simulink model "RemoteCHIL"  (Simulink 8.1)
settings: Solver=ode1  StartTime=0.0  StopTime=inf  FixedStep=Ts  MaxStep=1e-3  RelTol=1e-3
PostLoadFcn:
  | NREL_Mode=3; BANSHEE_init;
InitFcn:
  | NREL_Mode=3; BANSHEE_init;
values from neighbouring files (symbols this model uses):
  F4 = xlsread('F4_relay_nrel.xlsx')    [relay_settings_init.m]
  Ts = 100E-6    (= 0.0001)    [BANSHEE_init.m]    (also in Ghost_init.m)
undefined symbols (not defined in the file or in its folder): Left, Stim, type, V
libraries: simulink x50, relay_modbus_lib x11, simulink_extras x10, rtio_generic_modbus x6, rtlab x5, RMS_lib x4, cables_lib x3, relay_PLL_lib x3, PHIL_lib x2, breaker_lib x2, powerlib_extras x2, relay_ANSI_functions_lib x2
(part 2 of 3)

== system RemoteCHIL/SC_ctrl/TestSeq ==
  TestData : Inport
  Bias : Bias  Bias=[0:-1:-10]*1.1
  Bias1 : Bias  Bias=[0:-1:-2]*1.1
  Bias2 : Bias  Bias=[0:-1:-1]*1.1
  Bias3 : Bias  Bias=[0:-1:-1]*1.1
  Bus Selector : BusSelector  OutputSignals=TestSeq.seq_time,TestSeq.fault,TestSeq.dms,TestSeq.grid,TestSeq.motor,TestSeq.misc
  Bus Selector1 : BusSelector  OutputSignals=loc1,loc2,loc3,loc4,loc5,loc6,gen1,gen2,gen3,pv1,pv2  OutputAsBus=on
  Bus Selector2 : BusSelector  OutputSignals=DisReq,kWEna,PFEna  OutputAsBus=on
  Bus Selector3 : BusSelector  OutputSignals=kWref,PFref
  Bus Selector4 : BusSelector  OutputSignals=Dp,Dq  OutputAsBus=on
  Bus Selector5 : BusSelector  OutputSignals=Hz,Volt  OutputAsBus=on
  Bus Selector6 : BusSelector  OutputSignals=ena1,ena2  OutputAsBus=on
  Bus Selector7 : BusSelector  OutputSignals=cut_grid,mgc_ena  OutputAsBus=on
  Bus Selector8 : BusSelector  OutputSignals=TestSeq.price,TestSeq.pv.insolation1,TestSeq.pv.insolation2  OutputAsBus=on
  Display : Display
  Gain : Gain  Gain=[1/60 1/115000]
  TestSequence : Scope  NumInputPorts=9
      settings: YMin=-5~-5~-5~-5~-5~-5~-5~-5~-5  YMax=5~5~5~5~5~5~5~5~5  Decimation=50
  wires:
  TestData/1 -> Bus Selector8/1, Bus Selector/1
  Bus Selector/1 -> Display/1  "<seq_time>"
  Bus Selector/2 -> Bus Selector1/1  "<fault>"
  Bus Selector1/1 -> Bias/1
  Bias/1 -> TestSequence/1  "flt: loc1-6, gen1-3, ess1-2, pv1-2"
  Bus Selector2/1 -> Bias1/1
  Bias1/1 -> TestSequence/2  "dms: DisReq, kwCmd, PFCmd"
  Bus Selector3/1 -> TestSequence/3  "<kWref>"
  Bus Selector3/2 -> TestSequence/4  "<PFref>"
  Bus Selector4/1 -> TestSequence/5  "Dp, Dq"
  Bus Selector/3 -> Bus Selector3/1, Bus Selector4/1, Bus Selector2/1  "<dms>"
  Bus Selector/4 -> Bus Selector5/1  "<grid>"
  Bus Selector5/1 -> Gain/1
  Gain/1 -> TestSequence/6  "GridPU: Hz/Volt"
  Bus Selector/5 -> Bus Selector6/1  "<motor>"
  Bus Selector6/1 -> Bias2/1
  Bias2/1 -> TestSequence/7  "motor: ena1, ena2"
  Bus Selector/6 -> Bus Selector7/1  "<misc>"
  Bus Selector7/1 -> Bias3/1
  Bias3/1 -> TestSequence/8  "misc: cut_grid, mgc_ena"
  Bus Selector8/1 -> TestSequence/9  "price, pv1, pv2"

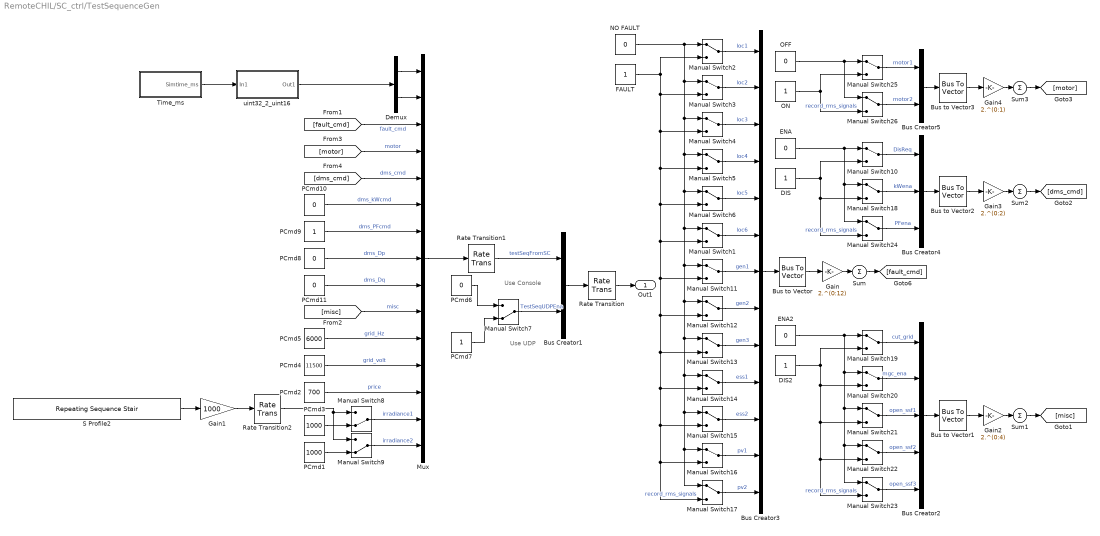
== system RemoteCHIL/SC_ctrl/TestSequenceGen ==
  note: Use Console
  note: Use UDP
  Bus Creator1 : BusCreator  Inputs=2
  Bus Creator2 : BusCreator  Inputs=5
  Bus Creator3 : BusCreator  Inputs=13
  Bus Creator4 : BusCreator  Inputs=3
  Bus Creator5 : BusCreator  Inputs=2
  Bus to Vector{,1..3} (4 alike) : BusToVector
  DIS : Constant
  DIS2 : Constant
  Demux : Demux  Outputs=2
  ENA : Constant  Value=0
  ENA2 : Constant  Value=0
  FAULT : Constant
  Gain : Gain  Gain=2.^(0:12)
  Gain1 : Gain  Gain=1000
  Gain2 : Gain  Gain=2.^(0:4)
  Gain3 : Gain  Gain=2.^(0:2)
  Gain4 : Gain  Gain=2.^(0:1)
  Manual Switch{1..6,10..26} (23 alike) : ManualSwitch
  Manual Switch7 : ManualSwitch  CurrentSetting=0
  Manual Switch8 : ManualSwitch  CurrentSetting=0
  Manual Switch9 : ManualSwitch  CurrentSetting=0
  Mux : Mux  Inputs=15
  NO FAULT : Constant  Value=0
  OFF : Constant  Value=0
  ON : Constant
  PCmd1 : Constant  Value=1000
  PCmd10 : Constant  Value=0
  PCmd11 : Constant  Value=0
  PCmd2 : Constant  Value=700
  PCmd3 : Constant  Value=1000
  PCmd4 : Constant  Value=11500
  PCmd5 : Constant  Value=6000
  PCmd6 : Constant  Value=0  SampleTime=[Stim.Ts Ts]
  PCmd7 : Constant
  PCmd8 : Constant  Value=0
  PCmd9 : Constant
  Rate Transition : RateTransition  Deterministic=off
  Rate Transition1 : RateTransition  Deterministic=off  OutPortSampleTime=1e-2
  Rate Transition2 : RateTransition  Deterministic=off  OutPortSampleTime=1e-2
  S Profile2 : simulink/Sources/Repeating Sequence Stair  OutValues=Stim.PV2.Irradiance  tsamp=[Stim.Ts Ts]  OutMin=[]  OutMax=[]  OutDataTypeStr=Inherit: Inherit via back propagation  OutDataType=fixdt(0,8)  ConRadixGroup=Best Precision: Vector-wise  OutScaling=2^-12
  Sum{,1..3} (4 alike) : Sum  Inputs=+
  Time_ms : Subsystem
  uint32_2_uint16 : Subsystem
      mask Display: disp('uint32_2_uint16');
  Out1 : Outport
  wires:
  Manual Switch4/1 -> Bus Creator3/3  "loc3"
  Manual Switch5/1 -> Bus Creator3/4  "loc4"
  [fault_cmd] -> Mux/3  "fault_cmd"
  Bus Creator3/1 -> Bus to Vector/1
  Manual Switch2/1 -> Bus Creator3/1  "loc1"
  Manual Switch6/1 -> Bus Creator3/5  "loc5"
  Manual Switch3/1 -> Bus Creator3/2  "loc2"
  Manual Switch1/1 -> Bus Creator3/6  "loc6"
  Manual Switch13/1 -> Bus Creator3/9  "gen3"
  Manual Switch14/1 -> Bus Creator3/10  "ess1"
  Manual Switch11/1 -> Bus Creator3/7  "gen1"
  Manual Switch15/1 -> Bus Creator3/11  "ess2"
  Manual Switch12/1 -> Bus Creator3/8  "gen2"
  FAULT/1 -> Manual Switch2/2, Manual Switch1/2, Manual Switch12/2, Manual Switch13/2, Manual Switch14/2, Manual Switch17/2, Manual Switch16/2, Manual Switch15/2, Manual Switch11/2, Manual Switch6/2, Manual Switch5/2, Manual Switch4/2, Manual Switch3/2  "record_rms_signals"
  NO FAULT/1 -> Manual Switch12/1, Manual Switch13/1, Manual Switch14/1, Manual Switch15/1, Manual Switch17/1, Manual Switch16/1, Manual Switch11/1, Manual Switch1/1, Manual Switch6/1, Manual Switch5/1, Manual Switch4/1, Manual Switch3/1, Manual Switch2/1
  Manual Switch16/1 -> Bus Creator3/12  "pv1"
  Manual Switch17/1 -> Bus Creator3/13  "pv2"
  Bus to Vector/1 -> Gain/1
  Gain/1 -> Sum/1
  Sum/1 -> [fault_cmd]
  Mux/1 -> Rate Transition1/1
  Bus Creator1/1 -> Rate Transition/1
  Manual Switch7/1 -> Bus Creator1/2  "TestSeqUDPEna"
  PCmd6/1 -> Manual Switch7/1
  PCmd7/1 -> Manual Switch7/2
  Rate Transition/1 -> Out1/1
  PCmd3/1 -> Manual Switch8/2
  Manual Switch9/1 -> Mux/15  "irradiance2"
  PCmd1/1 -> Manual Switch9/2
  Manual Switch8/1 -> Mux/14  "irradiance1"
  PCmd2/1 -> Mux/13  "price"
  Gain1/1 -> Rate Transition2/1
  Time_ms/1(Simtime_ms) -> uint32_2_uint16/1(In1)
  Demux/1 -> Mux/1
  Demux/2 -> Mux/2
  PCmd4/1 -> Mux/12  "grid_volt"
  PCmd5/1 -> Mux/11  "grid_Hz"
  [misc] -> Mux/10  "misc"
  [motor] -> Mux/4  "motor"
  [dms_cmd] -> Mux/5  "dms_cmd"
  PCmd8/1 -> Mux/8  "dms_Dp"
  PCmd9/1 -> Mux/7  "dms_PFcmd"
  PCmd10/1 -> Mux/6  "dms_kWcmd"
  PCmd11/1 -> Mux/9  "dms_Dq"
  Manual Switch21/1 -> Bus Creator2/3  "open_ssf1"
  Manual Switch22/1 -> Bus Creator2/4  "open_ssf2"
  Bus Creator2/1 -> Bus to Vector1/1
  Manual Switch19/1 -> Bus Creator2/1  "cut_grid"
  Manual Switch23/1 -> Bus Creator2/5  "open_ssf3"
  Manual Switch20/1 -> Bus Creator2/2  "mgc_ena"
  DIS2/1 -> Manual Switch20/2, Manual Switch21/2, Manual Switch22/2, Manual Switch23/2, Manual Switch19/2  "record_rms_signals"
  ENA2/1 -> Manual Switch19/1, Manual Switch20/1, Manual Switch21/1, Manual Switch22/1, Manual Switch23/1
  Bus to Vector1/1 -> Gain2/1
  Gain2/1 -> Sum1/1
  Sum1/1 -> [misc]
  Manual Switch24/1 -> Bus Creator4/3  "PFena"
  Bus Creator4/1 -> Bus to Vector2/1
  Manual Switch10/1 -> Bus Creator4/1  "DisReq"
  Manual Switch18/1 -> Bus Creator4/2  "kWena"
  DIS/1 -> Manual Switch10/2, Manual Switch24/2, Manual Switch18/2  "record_rms_signals"
  ENA/1 -> Manual Switch24/1, Manual Switch18/1, Manual Switch10/1
  Bus to Vector2/1 -> Gain3/1
  Gain3/1 -> Sum2/1
  Sum2/1 -> [dms_cmd]
  Bus Creator5/1 -> Bus to Vector3/1
  Manual Switch25/1 -> Bus Creator5/1  "motor1"
  Manual Switch26/1 -> Bus Creator5/2  "motor2"
  ON/1 -> Manual Switch26/2, Manual Switch25/2  "record_rms_signals"
  OFF/1 -> Manual Switch25/1, Manual Switch26/1
  Bus to Vector3/1 -> Gain4/1
  Gain4/1 -> Sum3/1
  Sum3/1 -> [motor]
  S Profile2/1 -> Gain1/1
  uint32_2_uint16/1(Out1) -> Demux/1
  Rate Transition1/1 -> Bus Creator1/1  "testSeqFromSC"
  Rate Transition2/1 -> Manual Switch9/1, Manual Switch8/1

== system RemoteCHIL/SS_F4_RELAY_HOUSING/BESS_data ==
  note: 0 .... 10000
      | 0 ... 100%
  Bus Selector1 : BusSelector  OutputSignals=Battery.SoC
  Bus Selector9 : BusSelector  OutputSignals=ESS_DATA
  Constant2 : Constant  Value=0
  Mux : Mux  Inputs=2
  Scale_SoC : Gain  Gain=100
  Out1 : Outport
  wires:
  Scale_SoC/1 -> Out1/1
  [F4_MS_IN] -> Bus Selector9/1
  Bus Selector9/1 -> Bus Selector1/1  "<ESS_DATA>"
  Bus Selector1/1 -> Mux/2  "<SoC>"
  Constant2/1 -> Mux/1
  Mux/1 -> Scale_SoC/1

== system RemoteCHIL/SS_F4_RELAY_HOUSING/DieselData ==
  Bus Selector : BusSelector  OutputSignals=GEN3_DATA.gen.gal_per_hr,GEN3_DATA.cb.relay_out.m.Vpu
  Constant1 : Constant  Value=0
  Constant4 : Constant  Value=0
  Mux : Mux
  scale_diesel1 : Gain  Gain=100
  scale_diesel2 : Gain  Gain=100
  Out2 : Outport
  wires:
  [F4_MS_IN] -> Bus Selector/1
  Bus Selector/1 -> scale_diesel1/1  "<gal_per_hr>"
  scale_diesel1/1 -> Mux/2
  Constant4/1 -> Mux/1
  Mux/1 -> Out2/1
  scale_diesel2/1 -> Mux/4
  Bus Selector/2 -> scale_diesel2/1  "<Vpu>"
  Constant1/1 -> Mux/3

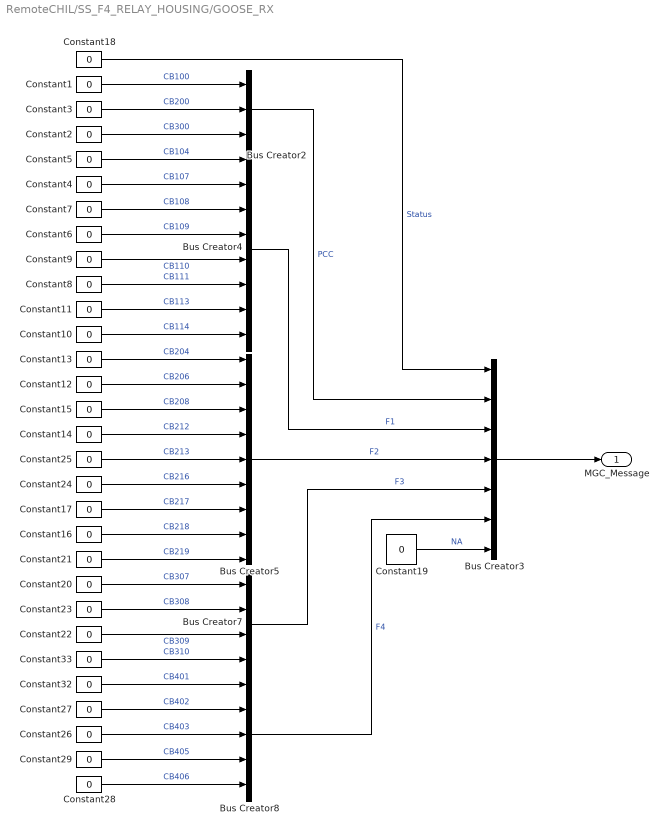
== system RemoteCHIL/SS_F4_RELAY_HOUSING/GOOSE_RX  ==
  Bus Creator2 : BusCreator  Inputs=3
  Bus Creator3 : BusCreator  Inputs=7
  Bus Creator4 : BusCreator  Inputs=8
  Bus Creator5 : BusCreator  Inputs=9
  Bus Creator7 : BusCreator
  Bus Creator8 : BusCreator  Inputs=5
  Constant{1..29,32..33} (31 alike) : Constant  Value=0
  MGC_Message : Outport
  wires:
  Constant18/1 -> Bus Creator3/1  "Status"
  Bus Creator3/1 -> MGC_Message/1
  Constant1/1 -> Bus Creator2/1  "CB100"
  Constant3/1 -> Bus Creator2/2  "CB200"
  Constant2/1 -> Bus Creator2/3  "CB300"
  Bus Creator2/1 -> Bus Creator3/2  "PCC"
  Constant7/1 -> Bus Creator4/3  "CB108"
  Constant6/1 -> Bus Creator4/4  "CB109"
  Constant4/1 -> Bus Creator4/2  "CB107"
  Constant9/1 -> Bus Creator4/5  "CB110"
  Constant5/1 -> Bus Creator4/1  "CB104"
  Constant8/1 -> Bus Creator4/6  "CB111"
  Constant11/1 -> Bus Creator4/7  "CB113"
  Constant10/1 -> Bus Creator4/8  "CB114"
  Bus Creator4/1 -> Bus Creator3/3  "F1"
  Constant21/1 -> Bus Creator5/9  "CB219"
  Constant24/1 -> Bus Creator5/6  "CB216"
  Constant17/1 -> Bus Creator5/7  "CB217"
  Constant25/1 -> Bus Creator5/5  "CB213"
  Constant16/1 -> Bus Creator5/8  "CB218"
  Constant15/1 -> Bus Creator5/3  "CB208"
  Constant13/1 -> Bus Creator5/1  "CB204"
  Constant14/1 -> Bus Creator5/4  "CB212"
  Constant12/1 -> Bus Creator5/2  "CB206"
  Bus Creator5/1 -> Bus Creator3/4  "F2"
  Bus Creator8/1 -> Bus Creator3/6  "F4"
  Constant28/1 -> Bus Creator8/5  "CB406"
  Constant26/1 -> Bus Creator8/3  "CB403"
  Bus Creator7/1 -> Bus Creator3/5  "F3"
  Constant33/1 -> Bus Creator7/4  "CB310"
  Constant22/1 -> Bus Creator7/3  "CB309"
  Constant23/1 -> Bus Creator7/2  "CB308"
  Constant20/1 -> Bus Creator7/1  "CB307"
  Constant19/1 -> Bus Creator3/7  "NA"
  Constant29/1 -> Bus Creator8/4  "CB405"
  Constant27/1 -> Bus Creator8/2  "CB402"
  Constant32/1 -> Bus Creator8/1  "CB401"

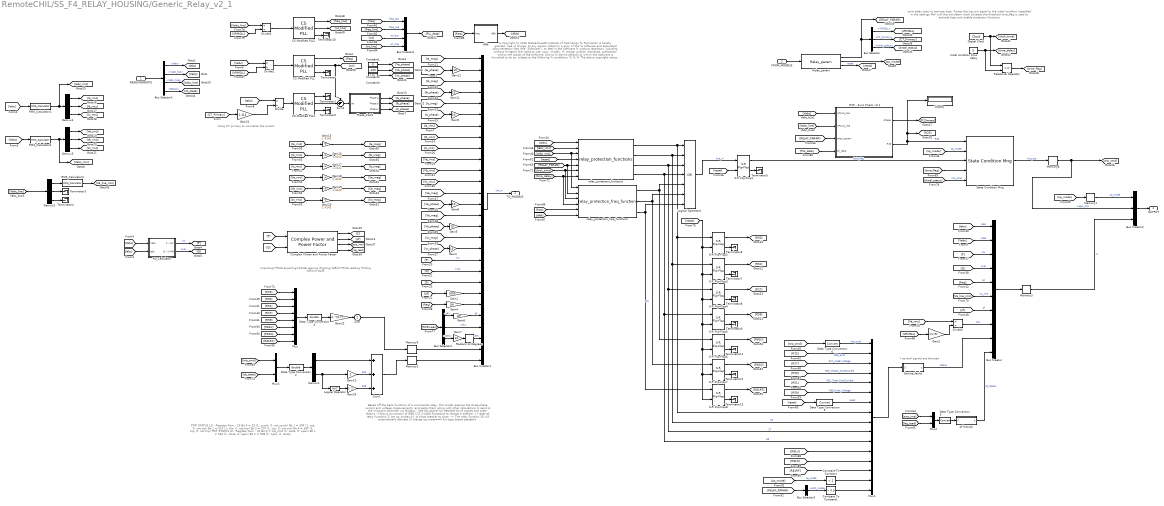
== system RemoteCHIL/SS_F4_RELAY_HOUSING/Generic_Relay_v2_1 ==
  note: time delay [sec] to activate logic. Forces the trip_out signal to the initial condition
      | (specified in the settings file) until the simulation clock exceeds the threshold
      |
      | time_flag is used to activate logic and enable protection functions
  note: Based off the basic functions of a commercial relay, this model receives
      | the three-phase current and voltage measurements, and packs
      | them along with other calculations to send to the microgrid
      | controller via Modbus
      |
      | - See HIL packet for detailed list of signals and scale factors
      | - Follows convention of IEEE C37.2-2008
      |
      | Procedure to reclose a breaker:
      | 1) reset all relay functions
      | 2) set op_mode==1 to force breaker to close
      |    --> The relay function 25 will automatically activate
      | 3) change op_mode==0 for logic based operation
  note: TRIP STATUS LO - Register Num.: 23
      | Bit 0 = 25  (1: synch, 0: not synch)
      | Bit 1 = 50P (1: trip, 0: not trip)
      | Bit 2 = 51P (1: trip, 0: not trip)
      | Bit 3 = 27P (1: trip, 0: not trip)
      | Bit 4 = 59P (1: trip, 0: not trip)
      |
      | TRIP STATUS HI - Register Num.: 24
      | Bit 0 = trip_cmd  (1: close, 0: open)
      | Bit 1 = 52A (1: close, 0: open)
      | Bit 2 = 52B (1: open, 0: close)
  note: Using CT primary to normalize the current.
  note: * several signals are bitwised
  note: Importing=TRUE
      | Exporting=FALSE
      |
      | Lagging (Pushing VARs)=TRUE
      | Leading (Pulling VARs)=FALSE
  note: % Copyright (c) 2016 Massachusetts Institute of Technology
      | % Permission is hereby granted, free of charge, to any person obtaining a copy of this
      | % software and associated documentation files (the "Software"), to deal in the Software
      | % without restriction, including without limitation the rights to use, copy, modify,
      | % merge, publish, distribute, sublicense, and/or sell copies of the Software, and to
      | % permit persons to whom the Software is furnished to do so, subject to the following
      | % conditions:
      | %
      | %
      | % The above copyright notice and this permission notice shall be included in
      | % all copies or substantial portions of the Software.
      | %
      | % THE SOFTWARE IS PROVIDED "AS IS", WITHOUT WARRANTY OF ANY KIND, EXPRESS OR IMPLIED,
      | % INCLUDING BUT NOT LIMITED TO THE WARRANTIES OF MERCHANTABILITY, FITNESS FOR A
      | % PARTICULAR PURPOSE AND NONINFRINGEMENT. IN NO EVENT SHALL THE AUTHORS OR COPYRIGHT
      | % HOLDERS BE LIABLE FOR ANY CLAIM, DAMAGES OR OTHER LIABILITY, WHETHER IN AN ACTION
      | % OF CONTRACT, TORT OR OTHERWISE, ARISING FROM, OUT OF OR IN CONNECTION WITH THE
      | % SOFTWARE OR THE USE OR OTHER DEALINGS IN THE SOFTWARE.
      | %
      | %
      | %%
  MEASUREMENTS : Inport
  FROM_MODBUS : Inport  Port=2
  Bus Creator : BusCreator  Inputs=10
  Bus Creator1 : BusCreator  Inputs=28
  Bus Creator2 : BusCreator  Inputs=3
  Bus Creator3 : BusCreator
  Bus Selector : BusSelector  OutputSignals=VRMSLL,CT_primary,Initial_status
  Bus Selector1 : BusSelector  OutputSignals=Iabc,Vabc_bus,Vabc_line,Status
  Bus Selector2 : BusSelector  OutputSignals=dF,dV,dWt
  Bus Selector3 : BusSelector  OutputSignals=prot_mode
  CS Modified PLL : relay_PLL_lib/CS Modified PLL  Flim=[55 66]  Par_Init=[0 60]  ParK=[ 180 3200 1 ]  Ts=Ts  AGC=off
  CS Modified PLL1 : relay_PLL_lib/CS Modified PLL  Flim=[55 66]  Par_Init=[0 60]  ParK=[ 180 3200 1 ]  Ts=Ts  AGC=off
  CS Modified PLL2 : relay_PLL_lib/CS Modified PLL  Flim=[55 66]  Par_Init=[0 60]  ParK=[ 180 3200 1 ]  Ts=Ts  AGC=off
  Compare To Constant : simulink/Logic and Bit Operations/Compare To Constant  relop=<  const=2  OutDataTypeStr=boolean
  Compare To Constant1 : simulink/Logic and Bit Operations/Compare To Constant  relop=>  const=0.5  OutDataTypeStr=boolean
  Complex Power and Power Factor : relay_PQSPF_lib/Complex Power and Power Factor
  Constant1 : Constant  Value=0
  Constant2 : Constant  Value=-120
  Constant3 : Constant  Value=120
  Data Type Conversion2 : DataTypeConversion  OutDataTypeStr=double
  Data Type Conversion3 : DataTypeConversion
  Data Type Conversion4 : DataTypeConversion  OutDataTypeStr=double
  Data Type Conversion5 : DataTypeConversion
  Data Type Conversion6 : DataTypeConversion
  Demux1 : Demux  Outputs=2
  Demux3 : Demux  Outputs=3
  Demux4 : Demux  Outputs=3
  Demux5 : Demux  Outputs=3
  Digital Clock : DigitalClock  SampleTime=Ts
  Display : Display
  Divide{,1..3} (4 alike) : Product  Inputs=*/
  Gain1 : Gain  Gain=1000
  Gain{3,5,7..9,11..12} (7 alike) : Gain  Gain=10
  Gain13 : Gain  Gain=2
  Gain{15..20} (6 alike) : Gain  Gain=1.4142
  Gain2 : Gain  Gain=1/1.732
  Gain21 : Gain  Gain=1.414
  Gain23 : Gain  Gain=2.^[0:7]
  Gain24 : Gain  Gain=2^2
  Gain4 : Gain  Gain=100
  Gain6 : Gain  Gain=100
  Logical Operator : Logic  Operator=NOT  AllPortsSameDT=off  OutDataTypeStr=boolean
  Logical Operator4 : Logic  Operator=OR  Inputs=7  AllPortsSameDT=off  OutDataTypeStr=boolean
  Memory{1..3,8..9} (5 alike) : Memory
  Mux : Mux  Inputs=8
  Mux1 : Mux  Inputs=16
  Mux2 : Mux  Inputs=2
  Mux3 : Mux  Inputs=2
  PQ_Calculator : Subsystem
  Phase_Calc1 : Subsystem
  R25 - Sync Check v0.1 : Subsystem  AncestorBlock=relay_ANSI_F25_lib/R25 - Sync Check v0.1  mask(Relay synch check){Ts=Ts}
      mask prompts: Ts "Sampling Time [Sec]"
      mask help:
      | This block checks if the the specified conditions for breaker reclosing
      | are met at both terminals of the circuit breaker. This synch check is
      | intended for use in bus-ties, and service lines.
      |
      | The input bus with the relay parameters should be ordered as follows:
      | 1) VRMSLL
      | 2) IOC
      | 3) TOC
      | 4) dV_threshold
      | 5) angle_threshold
      | 6) dF_threshold
  RMS_Calculator1 : RMS_lib/RMS_Calculator  Ts=Ts
  RMS_Calculator2 : RMS_lib/RMS_Calculator  Ts=Ts
  RMS_Calculator3 : RMS_lib/RMS_Calculator  Ts=Ts
  Radians to Degrees : simulink_extras/Transformations/Radians to Degrees
  Relational Operator : RelationalOperator  OutDataTypeStr=boolean
  Relay_param : relay_mgc_cmd_lib/Relay_param  relay_settings=relay_settings
  S-R Flip-Flop{1..8} (8 alike) : simulink_extras/Flip Flops/S-R Flip-Flop  initial_condition=0
  State Condition Mng : relay_tripOutMng_lib/State Condition Mng
  Sum : Sum  Inputs=+
  Sum1 : Sum  Inputs=+++
  Sum2 : Sum  Inputs=-+|
  Terminator{,1..13} (14 alike) : Terminator
  bitwise_faults : Subsystem
  dfdt : Subsystem
  initial condition time delay : Constant  Value=5
  pf bitwise : Subsystem
  relay_protection_freq_functions : relay_ANSI_functions_lib/relay_protection_freq_functions  Ts=Ts
  relay_protection_functions : relay_ANSI_functions_lib/relay_protection_functions  Ts=Ts
  OUTPUT : Outport
  TO_MODBUS : Outport  Port=2
  wires:
  Logical Operator4/1 -> S-R Flip-Flop1/1  "trip_in"
  [reset] -> S-R Flip-Flop1/2
  S-R Flip-Flop1/2 -> Terminator5/1
  Demux1/2 -> Gain13/1, Logical Operator/1
  Gain24/1 -> Sum1/3  "52B"
  [cb_state] -> Mux3/2
  [trip_cmd] -> Mux3/1
  Data Type Conversion2/1 -> Demux1/1
  Demux1/1 -> Sum1/1
  Gain13/1 -> Sum1/2  "52A"
  Mux3/1 -> Data Type Conversion2/1
  [R59] -> Mux/5
  [R27] -> Mux/4
  [R51] -> Mux/3
  [R50] -> Mux/2
  [R25] -> Mux/1
  Bus Selector1/4 -> [cb_state]  "<Status>"
  State Condition Mng/1 -> Memory8/1  "trip_out"
  Demux5/3 -> [Vc_rms]
  Demux5/2 -> [Vb_rms]
  Demux5/1 -> [Va_rms]
  Demux4/1 -> [Ia_rms]
  Demux4/2 -> [Ib_rms]
  Demux4/3 -> [Ic_rms]
  RMS_Calculator2/1 -> [Vabc_rms], Demux5/1
  RMS_Calculator1/1 -> [Iabc_rms], Demux4/1
  [Vabc] -> RMS_Calculator2/1
  [Iabc] -> RMS_Calculator1/1
  PQ_Calculator/2(Q - kVAR) -> [Q]  "kvar"
  PQ_Calculator/1(P - kW) -> [P]  "kw"
  [Iabc] -> PQ_Calculator/2(Iabc)
  [Vabc] -> PQ_Calculator/1(Vabc)
  [Iabc] -> Bus Creator/1  "Iabc"
  [Vabc] -> Bus Creator/2  "Vabc"
  FROM_MODBUS/1 -> Relay_param/1
  Bus Creator1/1 -> TO_MODBUS/1  "sm_in"
  [freq] -> Gain4/1
  [pf] -> Gain1/1
  [P] -> Bus Creator/3  "kw"
  [Q] -> Bus Creator/4  "kvar"
  Constant1/1 -> [Va_phase]
  Constant2/1 -> [Vb_phase]
  Constant3/1 -> [Vc_phase]
  [Iabc] -> Divide/1
  Phase_Calc1/1(Phase a) -> [Ia_phase]
  Phase_Calc1/2(Phase b) -> [Ib_phase]
  Phase_Calc1/3(Phase c) -> [Ic_phase]
  Divide/1 -> CS Modified PLL1/1
  [CT_Primary] -> Gain21/1
  [Vc_phase] -> Gain3/1
  [Vb_phase] -> Gain5/1
  [Va_phase] -> Gain8/1
  [Ic_phase] -> Gain9/1
  [Ib_phase] -> Gain11/1
  [Ia_phase] -> Gain12/1
  Sum1/1 -> Memory2/1
  Sum/1 -> Memory9/1
  relay_protection_functions/2 -> Mux1/9, S-R Flip-Flop3/1, Logical Operator4/2  "51"
  Mux/1 -> Data Type Conversion4/1
  Data Type Conversion4/1 -> Gain23/1
  Memory9/1 -> Bus Creator1/27
  Memory2/1 -> Bus Creator1/28
  [op_mode] -> Memory1/1
  Memory8/1 -> [trip_cmd], Bus Creator2/2  "Logic_trip"
  R25 - Sync Check v0.1/2(R25) -> Display/1, [R25], State Condition Mng/1  "R25"
  [op_mode] -> State Condition Mng/2  "op_mode"
  S-R Flip-Flop1/1 -> State Condition Mng/3  "fault_flag"
  CS Modified PLL1/2 -> Sum2/2
  CS Modified PLL/1 -> [freq]
  CS Modified PLL/2 -> [wt], Sum2/1
  CS Modified PLL1/1 -> Terminator1/1
  CS Modified PLL1/3 -> Terminator2/1
  CS Modified PLL/3 -> Terminator/1
  [freq] -> Bus Creator/5  "Hz"
  [Va_line_rms] -> Bus Creator/6  "Va_rms"
  [pf] -> Bus Creator/7  "pf"
  [Ia_mag] -> Bus Creator1/1
  Gain12/1 -> Bus Creator1/2
  [Ib_mag] -> Bus Creator1/3
  Gain11/1 -> Bus Creator1/4
  [Ic_mag] -> Bus Creator1/5
  Gain9/1 -> Bus Creator1/6
  [Ia_rms] -> Bus Creator1/7
  [Ib_rms] -> Bus Creator1/8
  [Ic_rms] -> Bus Creator1/9
  [Va_rms] -> Bus Creator1/10
  [Vb_rms] -> Bus Creator1/11
  [Vc_rms] -> Bus Creator1/12
  [Va_mag] -> Bus Creator1/13
  Gain8/1 -> Bus Creator1/14
  [Vb_mag] -> Bus Creator1/15
  Gain5/1 -> Bus Creator1/16
  [Vc_mag] -> Bus Creator1/17
  Gain3/1 -> Bus Creator1/18
  Gain1/1 -> Bus Creator1/22
  Gain4/1 -> Bus Creator1/23
  [Vabc] -> R25 - Sync Check v0.1/1(VPKLN_bus)
  [Ia_rms] -> Gain15/1
  [Ib_rms] -> Gain16/1
  [Ic_rms] -> Gain17/1
  [Va_rms] -> Gain18/1
  [Vb_rms] -> Gain19/1
  [Vc_rms] -> Gain20/1
  Gain20/1 -> [Vc_mag]
  Gain19/1 -> [Vb_mag]
  Gain18/1 -> [Va_mag]
  Gain17/1 -> [Ic_mag]
  Gain16/1 -> [Ib_mag]
  Gain15/1 -> [Ia_mag]
  Divide2/1 -> Bus Creator/8  "Vpu"
  relay_protection_functions/3 -> Mux1/10, S-R Flip-Flop4/1, Logical Operator4/3  "27"
  relay_protection_functions/4 -> Mux1/11, S-R Flip-Flop5/1, Logical Operator4/4  "59"
  Mux1/1 -> bitwise_faults/1(S)
  bitwise_faults/1(s) -> Bus Creator/9  "status"
  [reset] -> Data Type Conversion5/1
  [trip_cmd] -> Data Type Conversion6/1
  [R25] -> Mux1/2  "R25_Sync"
  [R27] -> Mux1/3  "R27_Under Voltage"
  [R50] -> Mux1/4  "R50_Instant_OverCurrent"
  [R51] -> Mux1/5  "R51_Time_OverCurrent"
  [R59] -> Mux1/6  "R59_Over_Voltage"
  Data Type Conversion5/1 -> Mux1/7  "reset"
  Data Type Conversion6/1 -> Mux1/1  "trip_cmd"
  [Vabc_line] -> R25 - Sync Check v0.1/2(VPKLN_line)
  Bus Selector1/1 -> [Iabc]  "<Iabc>"
  Bus Selector1/2 -> [Vabc]  "<Vabc_bus>"
  Bus Selector1/3 -> [Vabc_line]  "<Vabc_line>"
  MEASUREMENTS/1 -> Bus Selector1/1
  Bus Creator/1 -> Memory3/1
  Memory1/1 -> Bus Creator2/1  "op_mode"
  Bus Creator2/1 -> OUTPUT/1
  [P] -> Complex Power and Power Factor/1
  [Q] -> Complex Power and Power Factor/2
  Complex Power and Power Factor/1 -> [S]
  Complex Power and Power Factor/2 -> [pf]
  Complex Power and Power Factor/3 -> [exp_imp]
  Complex Power and Power Factor/4 -> [lag_lead]
  Mux2/1 -> Data Type Conversion3/1
  pf bitwise/1(s) -> Bus Creator/10  "pf_states"
  [exp_imp] -> Mux2/1
  [lag_lead] -> Mux2/2
  Memory3/1 -> Bus Creator2/3  "m"
  Data Type Conversion3/1 -> pf bitwise/1(S)
  Bus Selector/2 -> [CT_Primary]  "<CT_primary>"
  Relay_param/1 -> [RELAY_PARAM], Bus Selector/1
  [reset] -> relay_protection_functions/4
  [Iabc_rms] -> relay_protection_functions/2
  [Vabc_rms] -> relay_protection_functions/3, relay_protection_freq_functions/1
  [Iabc] -> relay_protection_functions/1
  [RELAY_PARAM] -> relay_protection_functions/5, relay_protection_freq_functions/2
  [RELAY_PARAM] -> R25 - Sync Check v0.1/3(relay_param)
  Bus Selector/1 -> [VRMSLL]  "<VRMSLL>"
  [Vabc] -> Divide1/1
  Divide1/1 -> CS Modified PLL/1
  [VRMSLL] -> Divide1/2
  [VRMSLL] -> Gain2/1
  [Va_rms] -> Divide2/1
  Relay_param/2 -> [op_mode]
  Gain21/1 -> Divide/2
  Digital Clock/1 -> Relational Operator/1, [clock_time]
  [time_flag] -> State Condition Mng/4
  initial condition time delay/1 -> Relational Operator/2, [time_delay]
  Relay_param/3 -> [reset]  "reset"
  [clock_time] -> relay_protection_functions/6, relay_protection_freq_functions/3
  [time_delay] -> relay_protection_functions/7, relay_protection_freq_functions/4
  Bus Selector/3 -> [Initial_status]  "<Initial_status>"
  [Initial_status] -> State Condition Mng/5  "init_cond"
  Logical Operator/1 -> Gain24/1
  Gain2/1 -> Divide2/2
  Demux3/1 -> RMS_Calculator3/1
  Demux3/2 -> Terminator3/1
  Demux3/3 -> Terminator4/1
  Relational Operator/1 -> [time_flag]
  [Vabc_line] -> Demux3/1
  RMS_Calculator3/1 -> [Va_line_rms]
  S-R Flip-Flop2/2 -> Terminator6/1
  S-R Flip-Flop3/2 -> Terminator7/1
  S-R Flip-Flop4/2 -> Terminator8/1
  S-R Flip-Flop5/2 -> Terminator9/1
  S-R Flip-Flop5/1 -> [R59]
  S-R Flip-Flop4/1 -> [R27]
  S-R Flip-Flop3/1 -> [R51]
  S-R Flip-Flop2/1 -> [R50]
  Sum2/1 -> Phase_Calc1/1(wt)
  [P] -> Bus Creator1/19  "kw"
  [Q] -> Bus Creator1/20  "kvar"
  [S] -> Bus Creator1/21
  relay_protection_functions/1 -> Mux1/8, S-R Flip-Flop2/1, Logical Operator4/1
  R25 - Sync Check v0.1/1(dMeas) -> [R25meas]
  [R25meas] -> Bus Selector2/1
  Bus Selector2/2 -> Bus Creator1/25  "<dV>"
  Bus Selector2/1 -> Gain6/1  "<dF>"
  Bus Selector2/3 -> Gain7/1  "<dWt>"
  Gain6/1 -> Bus Creator1/24  "dF"
  Gain7/1 -> Radians to Degrees/1
  Radians to Degrees/1 -> Bus Creator1/26  "dWt"
  [Vabc_line] -> Divide3/1
  [VRMSLL] -> Divide3/2
  Divide3/1 -> CS Modified PLL2/1
  CS Modified PLL2/1 -> [freq_line]
  CS Modified PLL2/2 -> [wt_line]
  CS Modified PLL2/3 -> Terminator10/1
  [PLL_data] -> R25 - Sync Check v0.1/4(pll_data)
  Bus Creator3/1 -> [PLL_data]
  [freq] -> Bus Creator3/1  "freq_bus"
  [freq_line] -> Bus Creator3/2  "freq_line"
  [wt] -> Bus Creator3/3  "wt_bus"
  [wt_line] -> Bus Creator3/4  "wt_line"
  [freq] -> dfdt/1(freq)
  dfdt/1(dfdt) -> [dfdt]
  [freq] -> relay_protection_freq_functions/5
  [dfdt] -> relay_protection_freq_functions/6
  relay_protection_freq_functions/3 -> S-R Flip-Flop8/1, Logical Operator4/7  "51"
  [reset] -> S-R Flip-Flop8/2, S-R Flip-Flop7/2, S-R Flip-Flop6/2, S-R Flip-Flop5/2, S-R Flip-Flop4/2, S-R Flip-Flop3/2, S-R Flip-Flop2/2
  S-R Flip-Flop6/2 -> Terminator11/1
  S-R Flip-Flop7/2 -> Terminator12/1
  S-R Flip-Flop8/2 -> Terminator13/1
  S-R Flip-Flop8/1 -> [R81RF]
  S-R Flip-Flop7/1 -> [R81O]
  S-R Flip-Flop6/1 -> [R81U]
  relay_protection_freq_functions/1 -> S-R Flip-Flop6/1, Logical Operator4/5
  relay_protection_freq_functions/2 -> Logical Operator4/6, S-R Flip-Flop7/1
  [R81U] -> Mux1/12
  [R81O] -> Mux1/13
  [R81RF] -> Mux1/14
  [op_mode] -> Compare To Constant/1  "op_mode"
  Compare To Constant/1 -> Mux1/15
  [RELAY_PARAM] -> Bus Selector3/1
  Bus Selector3/1 -> Compare To Constant1/1  "<prot_mode>"
  Compare To Constant1/1 -> Mux1/16
  [R81U] -> Mux/6
  [R81O] -> Mux/7
  [R81RF] -> Mux/8
  Gain23/1 -> Sum/1

== system RemoteCHIL/SS_F4_RELAY_HOUSING/MGC_controller ==
  Bus Selector1 : BusSelector  OutputSignals=GEN3_DATA,ESS_DATA,PV_DATA
  Bus Selector2 : BusSelector  OutputSignals=ctrl.raw
  Bus Selector3 : BusSelector  OutputSignals=raw
  Bus Selector4 : BusSelector  OutputSignals=raw
  Bus Selector5 : BusSelector  OutputSignals=F4_CB_CTRL  OutputAsBus=on
  Bus to Vector : BusToVector
  Constant : Constant  Value=zeros(1,14)
  Constant1 : Constant  Value=zeros(1,19)
  Constant2 : Constant  Value=zeros(1,10)
  Constant3 : Constant  Value=zeros(1,3)
  Constant{4..7} (4 alike) : Constant  Value=zeros(1,8)
  Vector Concatenate : Concatenate  NumInputs=12
  MGC_controller : Outport
  wires:
  Bus Selector4/1 -> Vector Concatenate/12  "<raw>"
  Constant7/1 -> Vector Concatenate/9
  Constant6/1 -> Vector Concatenate/8
  Constant5/1 -> Vector Concatenate/7
  Constant4/1 -> Vector Concatenate/6
  Bus Selector2/1 -> Vector Concatenate/10  "<raw>"
  Bus Selector3/1 -> Vector Concatenate/11  "<raw>"
  Bus Selector1/3 -> Bus Selector4/1  "<PV_DATA>"
  Bus Selector1/2 -> Bus Selector3/1  "<ESS_DATA>"
  Bus Selector1/1 -> Bus Selector2/1  "<GEN3_DATA>"
  [F4_MS_IN] -> Bus Selector1/1
  Constant2/1 -> Vector Concatenate/3
  Constant1/1 -> Vector Concatenate/2
  Constant/1 -> Vector Concatenate/1
  Constant3/1 -> Vector Concatenate/5
  Vector Concatenate/1 -> MGC_controller/1
  Bus to Vector/1 -> Vector Concatenate/4
  [F4_RELAY_OUT] -> Bus Selector5/1
  Bus Selector5/1 -> Bus to Vector/1

== system RemoteCHIL/SS_F4_RELAY_HOUSING/Misc_data ==
  note: Data ordered as:
      | I-P-C
      | kW-VRMSLL
  Bus Creator : BusCreator  Inputs=2
  Constant : Constant  Value=0
  Constant1 : Constant  Value=zeros(1,9)
  Mux8 : Mux  Inputs=2
  Mux9 : Mux  Inputs=2
  VRMSLL : Subsystem
  kW : Subsystem
  scale_load : Gain
  Out1 : Outport
  wires:
  scale_load/1 -> Mux9/1
  [F4_MS_IN] -> Bus Creator/1  "F4"
  Bus Creator/1 -> VRMSLL/1(In1), kW/1(In1)
  Mux8/1 -> scale_load/1
  Constant1/1 -> Mux9/2
  Mux9/1 -> Out1/1
  Constant/1 -> Bus Creator/2  "zero"
  kW/1(Out1) -> Mux8/1
  VRMSLL/1(Out1) -> Mux8/2

== system RemoteCHIL/SS_F4_RELAY_HOUSING/Power_quality_data ==
  Rst : Inport
  Bus Selector2 : BusSelector  OutputSignals=F4_CB_1.m.Vpu,F4_CB_2.m.Vpu,F4_CB_5.m.Vpu  OutputAsBus=on
  Bus Selector7 : BusSelector  OutputSignals=F4_CB_1.m.Hz,F4_CB_2.m.Hz,F4_CB_5.m.Hz  OutputAsBus=on
  Bus to Vector : BusToVector
  Bus to Vector3 : BusToVector
  Constant3 : Constant  Value=zeros(1,20)
  Constant4 : Constant  Value=zeros(1,20)
  IEEE1547a_Hz : power_quality_lib/IEEE1547a_Hz
  IEEE1547a_Volt : power_quality_lib/IEEE1547a_Hz
  Mux : Mux  Inputs=2
  Mux2 : Mux  Inputs=2
  Mux3 : Mux  Inputs=2
  Out1 : Outport
  wires:
  Bus to Vector3/1 -> IEEE1547a_Volt/1
  Bus Selector2/1 -> Bus to Vector3/1
  [F4_RELAY_OUT] -> Bus Selector7/1
  [F4_RELAY_OUT] -> Bus Selector2/1
  Constant3/1 -> Mux/1
  Bus to Vector/1 -> IEEE1547a_Hz/1
  Mux/1 -> Mux3/1
  Mux2/1 -> Mux3/2
  IEEE1547a_Volt/1 -> Mux2/2
  Mux3/1 -> Out1/1
  Constant4/1 -> Mux2/1
  Bus Selector7/1 -> Bus to Vector/1
  IEEE1547a_Hz/1 -> Mux/2
  Rst/1 -> IEEE1547a_Volt/2, IEEE1547a_Hz/2

== system RemoteCHIL/SS_F4_RELAY_HOUSING/Relay_data ==
  Constant : Constant  Value=zeros(1,14*5)
  Constant1 : Constant  Value=zeros(1,19*5)
  Constant2 : Constant  Value=zeros(1,10*5)
  Constant3 : Constant  Value=zeros(1,3*5)
  ExtractF4 : Subsystem
      mask Display: disp('Generic F4 relays\nID = 44 .. 49')
  Mux12 : Mux  Inputs=5
  Scale_freq2 : Gain  Gain=100
  Sel_freq : Selector  InputPortWidth=59*5  IndexOptions=Index vector (dialog)  Indices=[4:5:59*5]  OutputSizes=1
  Sel_kvar : Selector  InputPortWidth=59*5  IndexOptions=Index vector (dialog)  Indices=[2:5:59*5]  OutputSizes=1
  Sel_kw : Selector  InputPortWidth=59*5  IndexOptions=Index vector (dialog)  Indices=[1:5:59*5]  OutputSizes=1
  Sel_status : Selector  InputPortWidth=59*5  IndexOptions=Index vector (dialog)  Indices=[5:5:59*5]  OutputSizes=1
  Sel_vpu : Selector  InputPortWidth=59*5  IndexOptions=Index vector (dialog)  Indices=[3:5:59*5]  OutputSizes=1
  Subsystem1 : Subsystem
      mask Display: disp('GEN1,ESS1,PV1\nGEN2,GEN3,ESS2,PV1\nID = 53 .. 59')
  Vector Concatenate : Concatenate  NumInputs=6
  scale_kvar2 : Gain
  scale_kw2 : Gain
  scale_vpu2 : Gain  Gain=1000
  Out1 : Outport
  wires:
  [F4_RELAY_OUT] -> ExtractF4/1(In1)
  ExtractF4/1(Out1) -> Vector Concatenate/4
  Constant2/1 -> Vector Concatenate/3
  Constant1/1 -> Vector Concatenate/2
  Constant/1 -> Vector Concatenate/1
  Constant3/1 -> Vector Concatenate/5
  [F4_MS_IN] -> Subsystem1/1(F4)
  Subsystem1/1(Out1) -> Vector Concatenate/6
  Mux12/1 -> Out1/1
  scale_kw2/1 -> Mux12/1
  scale_kvar2/1 -> Mux12/2
  Scale_freq2/1 -> Mux12/4
  scale_vpu2/1 -> Mux12/3
  Sel_kw/1 -> scale_kw2/1
  Sel_status/1 -> Mux12/5
  Sel_freq/1 -> Scale_freq2/1
  Sel_vpu/1 -> scale_vpu2/1
  Sel_kvar/1 -> scale_kvar2/1
  Vector Concatenate/1 -> Sel_status/1, Sel_freq/1, Sel_vpu/1, Sel_kvar/1, Sel_kw/1

== system RemoteCHIL/SS_F4_RELAY_HOUSING/Time_ms ==
  Constant4 : Constant  Value=Ts/1e-3
  Sum : Sum  Inputs=++|
  Unit Delay : UnitDelay  SampleTime=-1
  Simtime_ms : Outport
  wires:
  Sum/1 -> Simtime_ms/1, Unit Delay/1
  Constant4/1 -> Sum/2
  Unit Delay/1 -> Sum/1

== system RemoteCHIL/SC_ctrl/CB_modbus_mock/F4 ==
  note: Op_Mode:
      | 0 = Relay Functions
      | 1 = Close Breaker
      | 2 = Open Breaker
  note: Copyright © 2017 the Alliance for Sustainable Energy, LLC
      |
      | The above copyright notice and this permission notice shall be included in all copies or substantial portions of the Software.
      |
      | THE SOFTWARE IS PROVIDED "AS IS", WITHOUT WARRANTY OF ANY KIND, EXPRESS OR IMPLIED, INCLUDING
      | BUT NOT LIMITED TO THE WARRANTIES OF MERCHANTABILITY, FITNESS FOR A PARTICULAR PURPOSE AND
      | NONINFRINGEMENT. IN NO EVENT SHALL THE AUTHORS OR COPYRIGHT HOLDERS BE LIABLE FOR ANY CLAIM,
      |  DAMAGES OR OTHER LIABILITY, WHETHER IN AN ACTION OF CONTRACT, TORT OR OTHERWISE, ARISING FROM,
      | OUT OF OR IN CONNECTION WITH THE SOFTWARE OR THE USE OR OTHER DEALINGS IN THE SOFTWARE
  Bus Creator3 : BusCreator  Inputs=6
  CB401 : simulink/Sources/Repeating Sequence Stair  OutValues=Stim.CB.CB401  tsamp=[Stim.Ts Ts]  OutMin=[]  OutMax=[]  OutDataTypeStr=Inherit: Inherit via back propagation  OutDataType=fixdt(0,8)  ConRadixGroup=Best Precision: Vector-wise  OutScaling=2^-12
  CB402 : simulink/Sources/Repeating Sequence Stair  OutValues=Stim.CB.CB402  tsamp=[Stim.Ts Ts]  OutMin=[]  OutMax=[]  OutDataTypeStr=Inherit: Inherit via back propagation  OutDataType=fixdt(0,8)  ConRadixGroup=Best Precision: Vector-wise  OutScaling=2^-12
  CB403 : simulink/Sources/Repeating Sequence Stair  OutValues=Stim.CB.CB403  tsamp=[Stim.Ts Ts]  OutMin=[]  OutMax=[]  OutDataTypeStr=Inherit: Inherit via back propagation  OutDataType=fixdt(0,8)  ConRadixGroup=Best Precision: Vector-wise  OutScaling=2^-12
  CB404 : simulink/Sources/Repeating Sequence Stair  OutValues=Stim.CB.CB404  tsamp=[Stim.Ts Ts]  OutMin=[]  OutMax=[]  OutDataTypeStr=Inherit: Inherit via back propagation  OutDataType=fixdt(0,8)  ConRadixGroup=Best Precision: Vector-wise  OutScaling=2^-12
  CB405 : simulink/Sources/Repeating Sequence Stair  OutValues=Stim.CB.CB405  tsamp=[Stim.Ts Ts]  OutMin=[]  OutMax=[]  OutDataTypeStr=Inherit: Inherit via back propagation  OutDataType=fixdt(0,8)  ConRadixGroup=Best Precision: Vector-wise  OutScaling=2^-12
  CB406 : simulink/Sources/Repeating Sequence Stair  OutValues=Stim.CB.CB406  tsamp=[Stim.Ts Ts]  OutMin=[]  OutMax=[]  OutDataTypeStr=Inherit: Inherit via back propagation  OutDataType=fixdt(0,8)  ConRadixGroup=Best Precision: Vector-wise  OutScaling=2^-12
  Constant{,1..5} (6 alike) : Constant  Value=0
  Manual Switch{1..6} (6 alike) : ManualSwitch
  Out1 : Outport
  wires:
  Bus Creator3/1 -> Out1/1  "F4"
  CB401/1 -> Manual Switch2/1
  Constant/1 -> Manual Switch2/2
  Manual Switch2/1 -> Bus Creator3/1  "CB401"
  Manual Switch6/1 -> Bus Creator3/6  "CB406"
  CB402/1 -> Manual Switch1/1
  Manual Switch1/1 -> Bus Creator3/2  "CB402"
  Manual Switch5/1 -> Bus Creator3/5  "CB405"
  Manual Switch3/1 -> Bus Creator3/3  "CB403"
  Manual Switch4/1 -> Bus Creator3/4  "CB404"
  Constant1/1 -> Manual Switch1/2
  CB403/1 -> Manual Switch3/1
  Constant2/1 -> Manual Switch3/2
  CB404/1 -> Manual Switch4/1
  Constant3/1 -> Manual Switch4/2
  CB405/1 -> Manual Switch5/1
  Constant4/1 -> Manual Switch5/2
  CB406/1 -> Manual Switch6/1
  Constant5/1 -> Manual Switch6/2

== system RemoteCHIL/SC_ctrl/ESS2 control/Tuning ==
  note: Not applicable
      | for PV
  Bus Creator : BusCreator  Inputs=7
  Constant : Constant  Value=2  SampleTime=[Stim.Ts Ts]
  Constant1 : Constant  Value=0.6e-3  SampleTime=[Stim.Ts Ts]
  Constant10 : Constant  Value=0  SampleTime=[Stim.Ts Ts]
  Constant2 : Constant  Value=180  SampleTime=[Stim.Ts Ts]
  Constant3 : Constant  Value=3200  SampleTime=[Stim.Ts Ts]
  Constant4 : Constant  SampleTime=[Stim.Ts Ts]
  Constant9 : Constant  SampleTime=[Stim.Ts Ts]
  Tuning : Outport
  wires:
  Bus Creator/1 -> Tuning/1
  Constant/1 -> Bus Creator/1  "csi_kp"
  Constant1/1 -> Bus Creator/2  "csi_Ti"
  Constant2/1 -> Bus Creator/3  "pll_kp"
  Constant3/1 -> Bus Creator/4  "pll_ki"
  Constant4/1 -> Bus Creator/5  "vff_ena"
  Constant10/1 -> Bus Creator/7  "batt_soc_rst"
  Constant9/1 -> Bus Creator/6  "batt_cap_div"

== system RemoteCHIL/SC_ctrl/PV2 control/Tuning ==
  note: Not applicable
      | for PV
  note: Nominal Insulation = 1000W/m^2
  note: A
      | --------
      | W/m^2
  Bus Creator : BusCreator  Inputs=13
  Constant : Constant  Value=2  SampleTime=[Stim.Ts Ts]
  Constant1 : Constant  Value=0.6e-3  SampleTime=[Stim.Ts Ts]
  Constant10 : Constant  SampleTime=[Stim.Ts Ts]
  Constant12 : Constant  Value=0.2
  Constant13 : Constant  Value=0
  Constant2 : Constant  Value=180  SampleTime=[Stim.Ts Ts]
  Constant3 : Constant  Value=3200  SampleTime=[Stim.Ts Ts]
  Constant4 : Constant  SampleTime=[Stim.Ts Ts]
  Constant5 : Constant  Value=31
  Constant6 : Constant  Value=36
  Constant7 : Constant
  Constant8 : Constant  Value=590
  Constant9 : Constant  SampleTime=[Stim.Ts Ts]
  Tuning : Outport
  wires:
  Constant4/1 -> Bus Creator/5  "vff_ena"
  Constant3/1 -> Bus Creator/4  "pll_ki"
  Constant2/1 -> Bus Creator/3  "pll_kp"
  Constant1/1 -> Bus Creator/2  "csi_Ti"
  Constant/1 -> Bus Creator/1  "csi_kp"
  Bus Creator/1 -> Tuning/1
  Constant6/1 -> Bus Creator/7  "ParallelN"
  Constant5/1 -> Bus Creator/6  "SeriesN"
  Constant7/1 -> Bus Creator/8  "Imin"
  Constant8/1 -> Bus Creator/9  "Vref"
  Constant10/1 -> Bus Creator/11  "batt_soc_rst"
  Constant9/1 -> Bus Creator/10  "batt_cap_div"
  Constant13/1 -> Bus Creator/12  "ConstCurEna"
  Constant12/1 -> Bus Creator/13  "ConstCurGain"

== system RemoteCHIL/SC_ctrl/Plots/status_bits_extract ==
  In1 : Inport
  Bias : Bias  Bias=[9:-1:0]*1.1
  Data Type Conversion : DataTypeConversion  OutDataTypeStr=uint16
  Data Type Conversion1 : DataTypeConversion  OutDataTypeStr=double
  Extract Bits1 : simulink/Logic and Bit Operations/Extract Bits  bitsToExtract=Range of bits  numBits=8  bitIdxRange=0  outScalingMode=Treat bit field as an integer
  Extract Bits10 : simulink/Logic and Bit Operations/Extract Bits  bitsToExtract=Range of bits  numBits=8  bitIdxRange=9  outScalingMode=Treat bit field as an integer
  Extract Bits2 : simulink/Logic and Bit Operations/Extract Bits  bitsToExtract=Range of bits  numBits=8  bitIdxRange=1  outScalingMode=Treat bit field as an integer
  Extract Bits3 : simulink/Logic and Bit Operations/Extract Bits  bitsToExtract=Range of bits  numBits=8  bitIdxRange=2  outScalingMode=Treat bit field as an integer
  Extract Bits4 : simulink/Logic and Bit Operations/Extract Bits  bitsToExtract=Range of bits  numBits=8  bitIdxRange=3  outScalingMode=Treat bit field as an integer
  Extract Bits5 : simulink/Logic and Bit Operations/Extract Bits  bitsToExtract=Range of bits  numBits=8  bitIdxRange=4  outScalingMode=Treat bit field as an integer
  Extract Bits6 : simulink/Logic and Bit Operations/Extract Bits  bitsToExtract=Range of bits  numBits=8  bitIdxRange=5  outScalingMode=Treat bit field as an integer
  Extract Bits7 : simulink/Logic and Bit Operations/Extract Bits  bitsToExtract=Range of bits  numBits=8  bitIdxRange=6  outScalingMode=Treat bit field as an integer
  Extract Bits8 : simulink/Logic and Bit Operations/Extract Bits  bitsToExtract=Range of bits  numBits=8  bitIdxRange=7  outScalingMode=Treat bit field as an integer
  Extract Bits9 : simulink/Logic and Bit Operations/Extract Bits  bitsToExtract=Range of bits  numBits=8  bitIdxRange=8  outScalingMode=Treat bit field as an integer
  Mux : Mux  Inputs=10
  Out1 : Outport
  wires:
  Bias/1 -> Out1/1
  Extract Bits5/1 -> Mux/5
  In1/1 -> Data Type Conversion/1
  Extract Bits2/1 -> Mux/2
  Data Type Conversion/1 -> Extract Bits1/1, Extract Bits2/1, Extract Bits3/1, Extract Bits4/1, Extract Bits5/1, Extract Bits8/1, Extract Bits10/1, Extract Bits9/1, Extract Bits7/1, Extract Bits6/1
  Mux/1 -> Data Type Conversion1/1
  Extract Bits1/1 -> Mux/1
  Data Type Conversion1/1 -> Bias/1
  Extract Bits10/1 -> Mux/10
  Extract Bits8/1 -> Mux/8
  Extract Bits9/1 -> Mux/9
  Extract Bits3/1 -> Mux/3
  Extract Bits4/1 -> Mux/4
  Extract Bits7/1 -> Mux/7
  Extract Bits6/1 -> Mux/6

== system RemoteCHIL/SC_ctrl/Plots/status_bits_extract1 ==
  In1 : Inport
  Bias : Bias  Bias=[9:-1:0]*1.1
  Data Type Conversion : DataTypeConversion  OutDataTypeStr=uint16
  Data Type Conversion1 : DataTypeConversion  OutDataTypeStr=double
  Extract Bits1 : simulink/Logic and Bit Operations/Extract Bits  bitsToExtract=Range of bits  numBits=8  bitIdxRange=0  outScalingMode=Treat bit field as an integer
  Extract Bits10 : simulink/Logic and Bit Operations/Extract Bits  bitsToExtract=Range of bits  numBits=8  bitIdxRange=9  outScalingMode=Treat bit field as an integer
  Extract Bits2 : simulink/Logic and Bit Operations/Extract Bits  bitsToExtract=Range of bits  numBits=8  bitIdxRange=1  outScalingMode=Treat bit field as an integer
  Extract Bits3 : simulink/Logic and Bit Operations/Extract Bits  bitsToExtract=Range of bits  numBits=8  bitIdxRange=2  outScalingMode=Treat bit field as an integer
  Extract Bits4 : simulink/Logic and Bit Operations/Extract Bits  bitsToExtract=Range of bits  numBits=8  bitIdxRange=3  outScalingMode=Treat bit field as an integer
  Extract Bits5 : simulink/Logic and Bit Operations/Extract Bits  bitsToExtract=Range of bits  numBits=8  bitIdxRange=4  outScalingMode=Treat bit field as an integer
  Extract Bits6 : simulink/Logic and Bit Operations/Extract Bits  bitsToExtract=Range of bits  numBits=8  bitIdxRange=5  outScalingMode=Treat bit field as an integer
  Extract Bits7 : simulink/Logic and Bit Operations/Extract Bits  bitsToExtract=Range of bits  numBits=8  bitIdxRange=6  outScalingMode=Treat bit field as an integer
  Extract Bits8 : simulink/Logic and Bit Operations/Extract Bits  bitsToExtract=Range of bits  numBits=8  bitIdxRange=7  outScalingMode=Treat bit field as an integer
  Extract Bits9 : simulink/Logic and Bit Operations/Extract Bits  bitsToExtract=Range of bits  numBits=8  bitIdxRange=8  outScalingMode=Treat bit field as an integer
  Mux : Mux  Inputs=10
  Out1 : Outport
  wires:
  Extract Bits6/1 -> Mux/6
  Extract Bits7/1 -> Mux/7
  Extract Bits4/1 -> Mux/4
  Extract Bits3/1 -> Mux/3
  Extract Bits9/1 -> Mux/9
  Extract Bits8/1 -> Mux/8
  Extract Bits10/1 -> Mux/10
  Data Type Conversion1/1 -> Bias/1
  Extract Bits1/1 -> Mux/1
  Mux/1 -> Data Type Conversion1/1
  Data Type Conversion/1 -> Extract Bits6/1, Extract Bits7/1, Extract Bits9/1, Extract Bits10/1, Extract Bits8/1, Extract Bits5/1, Extract Bits4/1, Extract Bits3/1, Extract Bits2/1, Extract Bits1/1
  Extract Bits2/1 -> Mux/2
  In1/1 -> Data Type Conversion/1
  Extract Bits5/1 -> Mux/5
  Bias/1 -> Out1/1

== system RemoteCHIL/SC_ctrl/TestSequenceGen/Time_ms ==
  Constant4 : Constant  Value=10
  Sum : Sum  Inputs=++|
  Unit Delay : UnitDelay  SampleTime=1e-2
  Simtime_ms : Outport
  wires:
  Unit Delay/1 -> Sum/1
  Constant4/1 -> Sum/2
  Sum/1 -> Unit Delay/1, Simtime_ms/1

== system RemoteCHIL/SC_ctrl/TestSequenceGen/uint32_2_uint16 ==
  In1 : Inport
  Data Type Conversion : DataTypeConversion  OutDataTypeStr=uint32
  Data Type Conversion1 : DataTypeConversion  OutDataTypeStr=double
  Data Type Conversion2 : DataTypeConversion  OutDataTypeStr=double
  Extract Bits : simulink/Logic and Bit Operations/Extract Bits  bitsToExtract=Upper half  numBits=8  bitIdxRange=[0 7]  outScalingMode=Treat bit field as an integer
  Extract Bits1 : simulink/Logic and Bit Operations/Extract Bits  bitsToExtract=Lower half  numBits=8  bitIdxRange=[0 7]  outScalingMode=Preserve fixed-point scaling
  Mux : Mux  Inputs=2
  Out1 : Outport
  wires:
  Extract Bits1/1 -> Data Type Conversion2/1
  Data Type Conversion1/1 -> Mux/2
  Data Type Conversion2/1 -> Mux/1
  Data Type Conversion/1 -> Extract Bits/1, Extract Bits1/1
  In1/1 -> Data Type Conversion/1
  Extract Bits/1 -> Data Type Conversion1/1
  Mux/1 -> Out1/1

== system RemoteCHIL/SS_F4_RELAY_HOUSING/Generic_Relay_v2_1/PQ_Calculator ==
  note: Copyright (c) 2016 Massachusetts Institute of Technology
      | Permission is hereby granted, free of charge, to any person obtaining a copy of this software and associated documentation files (the "Software"), to deal
      | in the Software without restriction, including without limitation the rights to use, copy, modify, merge, publish, distribute, sublicense, and/or sell copies of the
      | Software, and to permit persons to whom the Software is furnished to do so, subject to the following conditions:
      |
      | THE SOFTWARE IS PROVIDED "AS IS", WITHOUT WARRANTY OF ANY KIND, EXPRESS OR IMPLIED, INCLUDING BUT NOT LIMITED TO THE
      | WARRANTIES OF MERCHANTABILITY, FITNESS FOR A PARTICULAR PURPOSE AND NONINFRINGEMENT. IN NO EVENT SHALL THE AUTHORS
      | OR COPYRIGHT HOLDERS BE LIABLE FOR ANY CLAIM, DAMAGES OR OTHER LIABILITY, WHETHER IN AN ACTION OF CONTRACT, TORT OR
      | OTHERWISE, ARISING FROM, OUT OF OR IN CONNECTION WITH THE SOFTWARE OR THE USE OR OTHER DEALINGS IN THE SOFTWARE
  Vabc : Inport
  Iabc : Inport  Port=2
  3-phase  Instantaneous  Active & Reactive Power : powerlib_extras/Measurements/3-phase  Instantaneous  Active & Reactive Power
  Demux : Demux  Outputs=2
  Discrete  Mean value2 : powerlib_extras/Discrete Measurements/Discrete  Mean value  Freq=60  Vinit=0  Ts=Ts
  Gain10 : Gain  Gain=1/1000
  P - kW : Outport
  Q - kVAR : Outport  Port=2
  wires:
  Demux/2 -> Q - kVAR/1  "kvar"
  Demux/1 -> P - kW/1  "kw"
  Iabc/1 -> 3-phase  Instantaneous  Active & Reactive Power/2
  Vabc/1 -> 3-phase  Instantaneous  Active & Reactive Power/1
  Discrete  Mean value2/1 -> Gain10/1
  3-phase  Instantaneous  Active & Reactive Power/1 -> Discrete  Mean value2/1
  Gain10/1 -> Demux/1

== system RemoteCHIL/SS_F4_RELAY_HOUSING/Generic_Relay_v2_1/Phase_Calc1 ==
  note: Assumes Ib and Ic are shifted 120 degrees from Ia
      | For accurate phase measurements, could use a single-
      | phase PLL for each phase
  wt : Inport
  Add2 : Sum  Inputs=+-
  Add3 : Sum
  Constant5 : Constant  Value=120
  Constant6 : Constant  Value=120
  Constant7 : Constant  Value=360
  Constant8 : Constant  Value=360
  Gain : Gain  Gain=180/pi
  Math Function : Math  Operator=mod  SaturateOnIntegerOverflow=on
  Math Function1 : Math  Operator=mod  SaturateOnIntegerOverflow=on
  Phase a : Outport
  Phase b : Outport  Port=2
  Phase c : Outport  Port=3
  wires:
  Gain/1 -> Add2/1, Phase a/1, Add3/1
  Math Function1/1 -> Phase c/1
  Math Function/1 -> Phase b/1
  Constant8/1 -> Math Function1/2
  Add3/1 -> Math Function1/1
  Add2/1 -> Math Function/1
  Constant7/1 -> Math Function/2
  wt/1 -> Gain/1
  Constant6/1 -> Add3/2
  Constant5/1 -> Add2/2
